simulink model "ISTrain"  (R2024b)
settings: Solver=ode4  StartTime=0.0  StopTime=StopTime  FixedStep=StepSize  RelTol=1e-3
values from neighbouring files (symbols this model uses):
  Crr = 0.004    [run_ISTrain.m]
  eta_mech = 0.90    (= 0.9)    [run_ISTrain.m]
  g = 9.81    [run_ISTrain.m]
  G = 5    [run_ISTrain.m]
  grade = 0.02    [run_ISTrain.m]
  m_total = m_loco + m_trail    (= 2500)    [run_ISTrain.m]
  r_w = 0.100    (= 0.1)    [run_ISTrain.m]
settings Model: Creator=rafae  LastModifiedBy=rafae

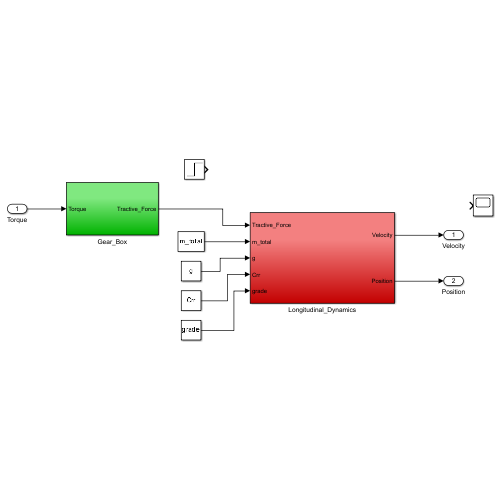
[thumbnail: Simulink's stored preview of the top-level diagram]
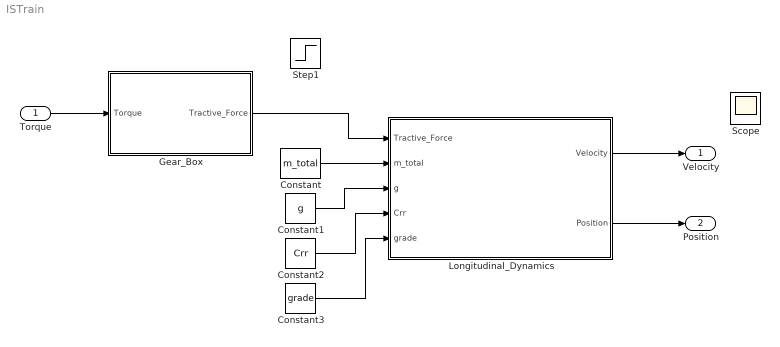
== system ISTrain ==
  Torque : Inport
  Constant : Constant  Value=m_total
  Constant1 : Constant  Value=g
  Constant2 : Constant  Value=Crr
  Constant3 : Constant  Value=grade
  Gear_Box : Subsystem
  Longitudinal_Dynamics : Subsystem
  Scope : Scope
  Step1 : Step  Time=100  After=130000  SampleTime=0
  Velocity : Outport
  Position : Outport  Port=2
  wires:
  Gear_Box/1(Tractive_Force) -> Longitudinal_Dynamics/1(Tractive_Force)
  Constant1/1 -> Longitudinal_Dynamics/3(g)
  Constant2/1 -> Longitudinal_Dynamics/4(Crr)
  Constant3/1 -> Longitudinal_Dynamics/5(grade)
  Longitudinal_Dynamics/1(Velocity) -> Velocity/1
  Longitudinal_Dynamics/2(Position) -> Position/1
  Constant/1 -> Longitudinal_Dynamics/2(m_total)
  Torque/1 -> Gear_Box/1(Torque)

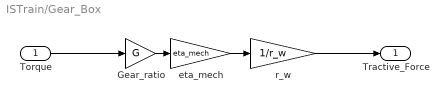
== system ISTrain/Gear_Box ==
  Torque : Inport
  Gear_ratio : Gain  Gain=G
  eta_mech : Gain  Gain=eta_mech
  r_w : Gain  Gain=1/r_w
  Tractive_Force : Outport
  wires:
  eta_mech/1 -> r_w/1
  Torque/1 -> Gear_ratio/1
  Gear_ratio/1 -> eta_mech/1
  r_w/1 -> Tractive_Force/1

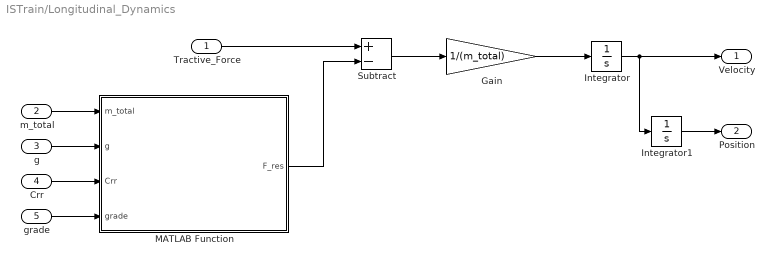
== system ISTrain/Longitudinal_Dynamics ==
  Tractive_Force : Inport
  m_total : Inport  Port=2
  g : Inport  Port=3
  Crr : Inport  Port=4
  grade : Inport  Port=5
  Gain : Gain  Gain=1/(m_total)
  Integrator : Integrator
  Integrator1 : Integrator
  MATLAB Function : MATLAB Function  TreatAsAtomicUnit=on
  Subtract : Sum  Inputs=+-
  Velocity : Outport
  Position : Outport  Port=2
  wires:
  Integrator1/1 -> Position/1
  Integrator/1 -> Velocity/1, Integrator1/1
  Gain/1 -> Integrator/1
  Tractive_Force/1 -> Subtract/1
  MATLAB Function/1(F_res) -> Subtract/2
  Crr/1 -> MATLAB Function/3(Crr)
  grade/1 -> MATLAB Function/4(grade)
  m_total/1 -> MATLAB Function/1(m_total)
  Subtract/1 -> Gain/1
  g/1 -> MATLAB Function/2(g)

== matlab function ISTrain/Longitudinal_Dynamics/MATLAB Function ==
  data: m_total input; F_res output; g input; Crr input; grade input
function F_res = ComputeResistance(m_total, g, Crr, grade)
F_rr = m_total * g * Crr;
F_grade = m_total * g * grade;
F_res = F_rr + F_grade;
end
